simulink library "GOcontroll_Moduline_Target"  (R2018b)
settings: Solver=ode45  StartTime=0.0  StopTime=10.0  RelTol=1e-3  EnableMultiTasking=on
(part 2 of 3)

== system GOcontroll_Moduline_Target/Modules/Input Module ==
  Input Module (10 channel) : Subsystem  Tag=HANcoder_GOcontroll_Moduline_IV  mask(Input Module){tsamp=0.1, ContrType=GOcontroll Moduline IV, moduleSlot=Moduleslot 1, SensSup1=Supply output enabled, C1func=Analog input -  decimal (12 bit resolution), C1pu=no pull up, C1pd=no pull down, C2func=Analog input -  decimal (12 bit resolution), C2pu=no pull up, C2pd=no pull down, C3func=Analog input -  decimal (12 bit resolution), C3pu=no pull up, C3pd=no pull down, C4func=Analog input -  decimal (12 bit resolution), C4pu=no pull up, C4pd=no pull down, C5func=Analog input -  decimal (12 bit resolution), C5pu=no pull up, C5pd=no pull down, C6func=Analog input -  decimal (12 bit resolution), C6pu=no pull up, C6pd=no pull down, C7func=Analog input -  decimal (12 bit resolution), C7pu=no pull up, C7pd=no pull down, C8func=Analog input -  decimal (12 bit resolution), C8pu=no pull up, C8pd=no pull down, C9func=Analog input -  decimal (12 bit resolution), C9pu=no pull up, C9pd=no pull down, C10func=Analog input -  decimal (12 bit resolution), C10pu=no pull up, C10pd=no pull down}
      mask prompts: tsamp "Sample time"; ContrType "Controller Type"; moduleSlot "Module Slot"; SensSup1 "5V Sensor Supply 1"; C1func "Function select"; C1pu "Pull up on input"; C1pd "Pull down on input"; C2func "Function select"; C2pu "Pull up on input"; C2pd "Pull down on input"; C3func "Function select"; C3pu "Pull up on input"; C3pd "Pull down on input"; C4func "Function select"; C4pu "Pull up on input"; C4pd "Pull down on input"; C5func "Function select"; C5pu "Pull up on input"; C5pd "Pull down on input"; C6func "Function select"; C6pu "Pull up on input"; C6pd "Pull down on input"; C7func "Function select"; C7pu "Pull up on input"; C7pd "Pull down on input"; C8func "Function select"; C8pu "Pull up on input"; C8pd "Pull down on input"; C9func "Function select"; C9pu "Pull up on input"; C9pd "Pull down on input"; C10func "Function select"; C10pu "Pull up on input"; C10pd "Pull down on input"
      mask help:
      | Whit this function block, you can configure each channel of the 6 channel input module (201001xx). The configuration of the module is executed once so the input module acts acording the setting. During runtime, the block outputs give the measured values from eacht measured channel which can directly be used inside the model.
      |
      | Module location:
      | Sets the location of the module slot where the module is physically
      | plugged into.
      |
      | Channel tabs:
      | Each channel has its own configuration tab.
      |
      | Function select:
      | Select the desired input signal configuration.
      |
      | Voltage range:
      | Select the expected input range of the signal.
      |
      | Analog filter samples:
      | The number of samples that are passed into a moving average filter.
      | (only active in case of an analog input)
      |
      | Pulses per rotation
      | The number of pulses for one rotation. This parameter is needed in case the
      | module needs to calculate the rotation speed from i.e. an axle.
      |
      | Pull Up:
      | If required, a pull-up resistance can be added to the input signal.
      |
      | Pull Down:
      | If required, a pull-down resistance can be added to the input signal.
      mask init:
      | [moduleSlotInfoStr, connectorId, pin1Id, pin2Id, pin3Id, pin4Id, pin5Id, pin6Id, pin7Id, pin8Id, pin9Id, pin10Id] = sfcn_gocontroll_input_module_10_mcb(moduleSlot,ContrType,C1func,C1pu,C1pd,...
      |                                                             C2func,C2pu,C2pd,...
      | 															C3func,C3pu,C3pd,...
      | 															C4func,C4pu,C4pd,...
      | 															C5func,C5pu,C5pd,...
      | 															C6func,C6pu,C6pd,...
      |                                                             C7func,C7pu,C7pd,...
      |                                                             C8func,C8pu,C8pd,...
      |                                                             C9func,C9pu,C9pd,...
      |                                                             C10func,C10pu,C10pd,...
      |                                                             SensSup1);
      settings: MoveFcn=%%drawLogos
      mask TypeOptions ContrType: GOcontroll Moduline IV | GOcontroll Moduline Mini | GOcontroll Moduline Display
      mask Callback ContrType:
      | msk = Simulink.Mask.get(gcb);
      | p = msk.Parameters;
      | 
      | func = get_param(gcb,'ContrType');
      | 
      | if(func == "GOcontroll Moduline IV")
      | p(3).TypeOptions = {'Moduleslot 1','Moduleslot 2','Moduleslot 3','Moduleslot 4',...
      |                     'Moduleslot 5','Moduleslot 6','Moduleslot 7','Moduleslot 8'};
      | elseif (func == "GOcontroll Moduline Mini")
      |  p(3).TypeOptions = {'Moduleslot 1','Moduleslot 2','Moduleslot 3','Moduleslot 4'};
      | 
      | else (func == "GOcontroll Moduline Screen")
      | p(3).TypeOptions = {'Moduleslot 1','Moduleslot 2'};
      | end
      mask TypeOptions moduleSlot: Moduleslot 1 | Moduleslot 2 | Moduleslot 3 | Moduleslot 4 | Moduleslot 5 | Moduleslot 6 | Moduleslot 7 | Moduleslot 8
      mask TypeOptions SensSup1: Supply output enabled | Supply output disabled
      mask TypeOptions C1func: Analog input -  decimal (12 bit resolution) | Analog input -  mV (1mV resolution) | Digital input - status (high or low) | Digital input - frequency (1Hz to 10 kHz) | Digital input - duty cycle low time (0.1% resolution) | Digital input - dutycycle high time (0.1% resolution) | Digital input - rotation speed (rpm) | Digital input - pulse counter (in combination with channel 2)
      mask TypeOptions C1pu: no pull up | 3,3 K ohm
      mask TypeOptions C1pd: no pull down | 3,3 K ohm
      mask TypeOptions C2func: Analog input -  decimal (12 bit resolution) | Analog input -  mV (1mV resolution) | Digital input - status (high or low) | Digital input - frequency (1Hz to 10 kHz) | Digital input - duty cycle low time (0.1% resolution) | Digital input - dutycycle high time (0.1% resolution) | Digital input - rotation speed (rpm) | Digital input - pulse counter (in combination with channel 2)
      mask TypeOptions C2pu: no pull up | 3,3 K ohm
      mask TypeOptions C2pd: no pull down | 3,3 K ohm
      mask TypeOptions C3func: Analog input -  decimal (12 bit resolution) | Analog input -  mV (1mV resolution) | Digital input - status (high or low) | Digital input - frequency (1Hz to 10 kHz) | Digital input - duty cycle low time (0.1% resolution) | Digital input - dutycycle high time (0.1% resolution) | Digital input - rotation speed (rpm) | Digital input - pulse counter (in combination with channel 2)
      mask TypeOptions C3pu: no pull up | 3,3 K ohm
      mask TypeOptions C3pd: no pull down | 3,3 K ohm
      mask TypeOptions C4func: Analog input -  decimal (12 bit resolution) | Analog input -  mV (1mV resolution) | Digital input - status (high or low) | Digital input - frequency (1Hz to 10 kHz) | Digital input - duty cycle low time (0.1% resolution) | Digital input - dutycycle high time (0.1% resolution) | Digital input - rotation speed (rpm) | Digital input - pulse counter (in combination with channel 2) | TFmini plus - Benewake LIDAR sensor
      mask TypeOptions C4pu: no pull up | 3,3 K ohm
      mask TypeOptions C4pd: no pull down | 3,3 K ohm
      mask TypeOptions C5func: Analog input -  decimal (12 bit resolution) | Analog input -  mV (1mV resolution) | Digital input - status (high or low) | Digital input - frequency (1Hz to 10 kHz) | Digital input - duty cycle low time (0.1% resolution) | Digital input - dutycycle high time (0.1% resolution) | Digital input - rotation speed (rpm) | Digital input - pulse counter (in combination with channel 2)
      mask TypeOptions C5pu: no pull up | 3,3 K ohm
      mask TypeOptions C5pd: no pull down | 3,3 K ohm
      mask TypeOptions C6func: Analog input -  decimal (12 bit resolution) | Analog input -  mV (1mV resolution) | Digital input - status (high or low) | Digital input - frequency (1Hz to 10 kHz) | Digital input - duty cycle low time (0.1% resolution) | Digital input - dutycycle high time (0.1% resolution) | Digital input - rotation speed (rpm) | Digital input - pulse counter (in combination with channel 2)
      mask TypeOptions C6pu: no pull up | 3,3 K ohm
      mask TypeOptions C6pd: no pull down | 3,3 K ohm
      mask TypeOptions C7func: Analog input -  decimal (12 bit resolution) | Analog input -  mV (1mV resolution) | Digital input - status (high or low) | Digital input - frequency (1Hz to 10 kHz) | Digital input - duty cycle low time (0.1% resolution) | Digital input - dutycycle high time (0.1% resolution) | Digital input - rotation speed (rpm) | Digital input - pulse counter (in combination with channel 2)
      mask TypeOptions C7pu: no pull up | 3,3 K ohm
      mask TypeOptions C7pd: no pull down | 3,3 K ohm
      mask TypeOptions C8func: Analog input -  decimal (12 bit resolution) | Analog input -  mV (1mV resolution) | Digital input - status (high or low) | Digital input - frequency (1Hz to 10 kHz) | Digital input - duty cycle low time (0.1% resolution) | Digital input - dutycycle high time (0.1% resolution) | Digital input - rotation speed (rpm) | Digital input - pulse counter (in combination with channel 2)
      mask TypeOptions C8pu: no pull up | 3,3 K ohm
      mask TypeOptions C8pd: no pull down | 3,3 K ohm
      mask TypeOptions C9func: Analog input -  decimal (12 bit resolution) | Analog input -  mV (1mV resolution) | Digital input - status (high or low) | Digital input - frequency (1Hz to 10 kHz) | Digital input - duty cycle low time (0.1% resolution) | Digital input - dutycycle high time (0.1% resolution) | Digital input - rotation speed (rpm) | Digital input - pulse counter (in combination with channel 2) | TFmini plus - Benewake LIDAR sensor
      mask TypeOptions C9pu: no pull up | 3,3 K ohm
      mask TypeOptions C9pd: no pull down | 3,3 K ohm
      mask TypeOptions C10func: Analog input -  decimal (12 bit resolution) | Analog input -  mV (1mV resolution) | Digital input - status (high or low) | Digital input - frequency (1Hz to 10 kHz) | Digital input - duty cycle low time (0.1% resolution) | Digital input - dutycycle high time (0.1% resolution) | Digital input - rotation speed (rpm) | Digital input - pulse counter (in combination with channel 2)
      mask TypeOptions C10pu: no pull up | 3,3 K ohm
      mask TypeOptions C10pd: no pull down | 3,3 K ohm
      mask DialogControl Container4 Prompt: Input 1
      mask DialogControl Container5 Prompt: Input 2
      mask DialogControl Container8 Prompt: Input 3
      mask DialogControl Container9 Prompt: Input 4
      mask DialogControl Container7 Prompt: Input 5
      mask DialogControl Container12 Prompt: Input 6
      mask DialogControl Container6 Prompt: Input 7
      mask DialogControl Container10 Prompt: Input 8
      mask DialogControl Container11 Prompt: Input 9
      mask DialogControl Container13 Prompt: Input 10
      mask Display:
      | fprintf('10 Channel Input Module \n%s\n\n Controller Connector: %s', moduleSlotInfoStr,connectorId);
      | port_label('output', 1, pin1Id);
      | port_label('output', 2, pin2Id);
      | port_label('output', 3, pin3Id);
      | port_label('output', 4, pin4Id);
      | port_label('output', 5, pin5Id);
      | port_label('output', 6, pin6Id);
      | port_label('output', 7, pin7Id);
      | port_label('output', 8, pin8Id);
      | port_label('output', 9, pin9Id);
      | port_label('output', 10, pin10Id);
      | text(2, 6, ert_linux_target_version());
  Input Module (6 channel) : Subsystem  Tag=HANcoder_GOcontroll_Moduline_IV  mask(Input Module){tsamp=0.1, ContrType=GOcontroll Moduline IV, moduleSlot=Moduleslot 1, SensSup1=Supply output enabled, SensSup2=Supply output enabled, SensSup3=Supply output enabled, C1func=Analog input -  decimal (12 bit resolution), C1volt=0 - 5 V, C1afil=0, C1dpul=1, C1pu=no pull up, C1pd=no pull down, C2func=Analog input -  decimal (12 bit resolution), C2volt=0 - 5 V, C2afil=0, C2dpul=1, C2pu=no pull up, C2pd=no pull down, C3func=Analog input -  decimal (12 bit resolution), C3volt=0 - 5 V, C3afil=0, C3dpul=1, C3pu=no pull up, C3pd=no pull down, C4func=Analog input -  decimal (12 bit resolution), C4volt=0 - 5 V, C4afil=0, C4dpul=1, C4pu=no pull up, C4pd=no pull down, C5func=Analog input -  decimal (12 bit resolution), C5volt=0 - 5 V, C5afil=0, C5dpul=1, C5pu=no pull up, C5pd=no pull down, C6func=Analog input -  decimal (12 bit resolution), C6volt=0 - 5 V, C6afil=0, C6dpul=1, C6pu=no pull up, C6pd=no pull down}
      mask prompts: tsamp "Sample time"; ContrType "Controller Type"; moduleSlot "Module Slot"; SensSup1 "5V Sensor Supply 1"; SensSup2 "5V Sensor Supply 2"; SensSup3 "5V Sensor Supply 3"; C1func "Function select"; C1volt "Voltage range"; C1afil "Analog filter samples (0 - 1000)"; C1dpul "Pulses per rotation (1-200)"; C1pu "Pull up on input"; C1pd "Pull down on input"; C2func "Function select"; C2volt "Voltage range"; C2afil "Analog filter samples (0 - 1000)"; C2dpul "Pulses per rotation (1-200)"; C2pu "Pull up on input"; C2pd "Pull down on input"; C3func "Function select"; C3volt "Voltage range"; C3afil "Analog filter samples (0 - 1000)"; C3dpul "Pulses per rotation (1-200)"; C3pu "Pull up on input"; C3pd "Pull down on input"; C4func "Function select"; C4volt "Voltage range"; C4afil "Analog filter samples (0 - 1000)"; C4dpul "Pulses per rotation (1-200)"; C4pu "Pull up on input"; C4pd "Pull down on input"; C5func "Function select"; C5volt "Voltage range"; C5afil "Analog filter samples (0 - 1000)"; C5dpul "Pulses per rotation (1-200)"; C5pu "Pull up on input"; C5pd "Pull down on input"; C6func "Function select"; C6volt "Voltage range"; C6afil "Analog filter samples (0 - 1000)"; C6dpul "Pulses per rotation (1-200)"; C6pu "Pull up on input"; C6pd "Pull down on input"
      mask help:
      | Whit this function block, you can configure each channel of the 6 channel input module (201001xx). The configuration of the module is executed once so the input module acts acording the setting. During runtime, the block outputs give the measured values from eacht measured channel which can directly be used inside the model.
      |
      | Module location:
      | Sets the location of the module slot where the module is physically
      | plugged into.
      |
      | Channel tabs:
      | Each channel has its own configuration tab.
      |
      | Function select:
      | Select the desired input signal configuration.
      |
      | Voltage range:
      | Select the expected input range of the signal.
      |
      | Analog filter samples:
      | The number of samples that are passed into a moving average filter.
      | (only active in case of an analog input)
      |
      | Pulses per rotation
      | The number of pulses for one rotation. This parameter is needed in case the
      | module needs to calculate the rotation speed from i.e. an axle.
      |
      | Pull Up:
      | If required, a pull-up resistance can be added to the input signal.
      |
      | Pull Down:
      | If required, a pull-down resistance can be added to the input signal.
      mask init:
      | [moduleSlotInfoStr, connectorId, pin1Id, pin2Id, pin3Id, pin4Id, pin5Id, pin6Id] = sfcn_gocontroll_input_module_mcb(moduleSlot,ContrType, C1func,C1volt,C1afil,C1dpul,C1pu,C1pd,...
      |                                                             C2func,C2volt,C2afil,C2dpul,C2pu,C2pd,...
      | 															C3func,C3volt,C3afil,C3dpul,C3pu,C3pd,...
      | 															C4func,C4volt,C4afil,C4dpul,C4pu,C4pd,...
      | 															C5func,C5volt,C5afil,C5dpul,C5pu,C5pd,...
      | 															C6func,C6volt,C6afil,C6dpul,C6pu,C6pd,...
      |                                                             SensSup1,SensSup2,SensSup3);
      settings: MoveFcn=%%drawLogos
      mask TypeOptions ContrType: GOcontroll Moduline IV | GOcontroll Moduline Mini | GOcontroll Moduline Display
      mask Callback ContrType:
      | msk = Simulink.Mask.get(gcb);
      | p = msk.Parameters;
      | 
      | func = get_param(gcb,'ContrType');
      | 
      | if(func == "GOcontroll Moduline IV")
      | p(3).TypeOptions = {'Moduleslot 1','Moduleslot 2','Moduleslot 3','Moduleslot 4',...
      |                     'Moduleslot 5','Moduleslot 6','Moduleslot 7','Moduleslot 8'};
      | elseif (func == "GOcontroll Moduline Mini")
      |  p(3).TypeOptions = {'Moduleslot 1','Moduleslot 2','Moduleslot 3','Moduleslot 4'};
      | 
      | else (func == "GOcontroll Moduline Screen")
      | p(3).TypeOptions = {'Moduleslot 1','Moduleslot 2'};
      | end
      mask TypeOptions moduleSlot: Moduleslot 1 | Moduleslot 2 | Moduleslot 3 | Moduleslot 4 | Moduleslot 5 | Moduleslot 6 | Moduleslot 7 | Moduleslot 8
      mask TypeOptions SensSup1: Supply output enabled | Supply output disabled
      mask TypeOptions SensSup2: Supply output enabled | Supply output disabled
      mask TypeOptions SensSup3: Supply output enabled | Supply output disabled
      mask TypeOptions C1func: Analog input -  decimal (12 bit resolution) | Analog input -  mV (1mV resolution) | Digital input - status (high or low) | Digital input - frequency (1Hz to 10 kHz) | Digital input - duty cycle low time (0.1% resolution) | Digital input - dutycycle high time (0.1% resolution) | Digital input - rotation speed (rpm) | Digital input - pulse counter (in combination with channel 2)
      mask TypeOptions C1volt: 0 - 5 V | 0 - 10V (external sensor supply) | 0 - 24V (external sensor supply)
      mask TypeOptions C1pu: no pull up | 3,3 K ohm | 4,7 K ohm | 10 K ohm
      mask TypeOptions C1pd: no pull down | 3,3 K ohm | 4,7 K ohm | 10 K ohm
      mask TypeOptions C2func: Analog input -  decimal (12 bit resolution) | Analog input -  mV (1mV resolution) | Digital input - status (high or low) | Digital input - frequency (1Hz to 10 kHz) | Digital input - duty cycle low time (0.1% resolution) | Digital input - dutycycle high time (0.1% resolution) | Digital input - rotation speed (rpm) | Digital input - pulse counter (in combination with channel 2)
      mask TypeOptions C2volt: 0 - 5 V | 0 - 10V (external sensor supply) | 0 - 24V (external sensor supply)
      mask TypeOptions C2pu: no pull up | 3,3 K ohm | 4,7 K ohm | 10 K ohm
      mask TypeOptions C2pd: no pull down | 3,3 K ohm | 4,7 K ohm | 10 K ohm
      mask TypeOptions C3func: Analog input -  decimal (12 bit resolution) | Analog input -  mV (1mV resolution) | Digital input - status (high or low) | Digital input - frequency (1Hz to 10 kHz) | Digital input - duty cycle low time (0.1% resolution) | Digital input - dutycycle high time (0.1% resolution) | Digital input - rotation speed (rpm) | Digital input - pulse counter (in combination with channel 2)
      mask TypeOptions C3volt: 0 - 5 V | 0 - 10V (external sensor supply) | 0 - 24V (external sensor supply)
      mask TypeOptions C3pu: no pull up | 3,3 K ohm | 4,7 K ohm | 10 K ohm
      mask TypeOptions C3pd: no pull down | 3,3 K ohm | 4,7 K ohm | 10 K ohm
      mask TypeOptions C4func: Analog input -  decimal (12 bit resolution) | Analog input -  mV (1mV resolution) | Digital input - status (high or low) | Digital input - frequency (1Hz to 10 kHz) | Digital input - duty cycle low time (0.1% resolution) | Digital input - dutycycle high time (0.1% resolution) | Digital input - rotation speed (rpm) | Digital input - pulse counter (in combination with channel 2) | TFmini plus - Benewake LIDAR sensor
      mask TypeOptions C4volt: 0 - 5 V | 0 - 10V (external sensor supply) | 0 - 24V (external sensor supply)
      mask TypeOptions C4pu: no pull up | 3,3 K ohm | 4,7 K ohm | 10 K ohm
      mask TypeOptions C4pd: no pull down | 3,3 K ohm | 4,7 K ohm | 10 K ohm
      mask TypeOptions C5func: Analog input -  decimal (12 bit resolution) | Analog input -  mV (1mV resolution) | Digital input - status (high or low) | Digital input - frequency (1Hz to 10 kHz) | Digital input - duty cycle low time (0.1% resolution) | Digital input - dutycycle high time (0.1% resolution) | Digital input - rotation speed (rpm) | Digital input - pulse counter (in combination with channel 2)
      mask TypeOptions C5volt: 0 - 5 V | 0 - 10V (external sensor supply) | 0 - 24V (external sensor supply)
      mask TypeOptions C5pu: no pull up | 3,3 K ohm | 4,7 K ohm | 10 K ohm
      mask TypeOptions C5pd: no pull down | 3,3 K ohm | 4,7 K ohm | 10 K ohm
      mask TypeOptions C6func: Analog input -  decimal (12 bit resolution) | Analog input -  mV (1mV resolution) | Digital input - status (high or low) | Digital input - frequency (1Hz to 10 kHz) | Digital input - duty cycle low time (0.1% resolution) | Digital input - dutycycle high time (0.1% resolution) | Digital input - rotation speed (rpm) | Digital input - pulse counter (in combination with channel 2)
      mask TypeOptions C6volt: 0 - 5 V | 0 - 10V (external sensor supply) | 0 - 24V (external sensor supply)
      mask TypeOptions C6pu: no pull up | 3,3 K ohm | 4,7 K ohm | 10 K ohm
      mask TypeOptions C6pd: no pull down | 3,3 K ohm | 4,7 K ohm | 10 K ohm
      mask DialogControl Container4 Prompt: Input 1
      mask DialogControl Container5 Prompt: Input 2
      mask DialogControl Container8 Prompt: Input 3
      mask DialogControl Container9 Prompt: Input 4
      mask DialogControl Container7 Prompt: Input 5
      mask DialogControl Container12 Prompt: Input 6
      mask Display:
      | fprintf('6 Channel Input Module \n%s\n\n Controller Connector: %s', moduleSlotInfoStr,connectorId);
      | port_label('output', 1, pin1Id);
      | port_label('output', 2, pin2Id);
      | port_label('output', 3, pin3Id);
      | port_label('output', 4, pin4Id);
      | port_label('output', 5, pin5Id);
      | port_label('output', 6, pin6Id);
      | text(2, 6, ert_linux_target_version());
  Input Module 4-20 mA (10 channel) : Subsystem  Tag=HANcoder_GOcontroll_Moduline_IV  mask(4-20 mA Input Module){tsamp=0.1, ContrType=GOcontroll Moduline IV, moduleSlot=Moduleslot 1, Sup16va=Supply enabled}
      mask prompts: tsamp "Sample time"; ContrType "Controller type"; moduleSlot "Module slot"; Sup16va "16V sensor supply"
      mask help:
      | Controller type:
      | Selects the controller that is to be programmed. Pinning on the mask will be adopted accordingly.
      |
      | Module slot:
      | Sets the location of the module slot where the module is physically plugged into.
      |
      | 16V sensor supply:
      | Enables the 16V supply for all the sensors. When this supply is not enabled possible no current flows through the sensors.
      |
      | Module status:
      | The status output provides information of the actual state per 2 channels:
      | 0x00 all channels are supplied no problems.
      | 0x01Channel 1 & 2 over current detected and supply disconnected.
      | 0x02Channel 3 & 4 over current detected and supply disconnected.
      | 0x04Channel 5 & 6 over current detected and supply disconnected.
      | 0x08Channel 7 & 8 over current detected and supply disconnected.
      | 0x10Channel 9 & 10 over current detected and supply disconnected.
      mask init:
      | [moduleSlotInfoStr, connectorId, pin1Id, pin2Id, pin3Id, pin4Id, pin5Id, pin6Id, pin7Id, pin8Id, pin9Id, pin10Id] =...
      |     sfcn_gocontroll_input_module_420ma_mcb(moduleSlot,ContrType,Sup16va);
      settings: MoveFcn=%%drawLogos
      mask TypeOptions ContrType: GOcontroll Moduline IV | GOcontroll Moduline Mini | GOcontroll Moduline Display
      mask Callback ContrType:
      | msk = Simulink.Mask.get(gcb);
      | p = msk.Parameters;
      | 
      | func = get_param(gcb,'ContrType');
      | 
      | if(func == "GOcontroll Moduline IV")
      | p(3).TypeOptions = {'Moduleslot 1','Moduleslot 2','Moduleslot 3','Moduleslot 4',...
      |                     'Moduleslot 5','Moduleslot 6','Moduleslot 7','Moduleslot 8'};
      | elseif (func == "GOcontroll Moduline Mini")
      |  p(3).TypeOptions = {'Moduleslot 1','Moduleslot 2','Moduleslot 3','Moduleslot 4'};
      | 
      | else (func == "GOcontroll Moduline Screen")
      | p(3).TypeOptions = {'Moduleslot 1','Moduleslot 2'};
      | end
      mask TypeOptions moduleSlot: Moduleslot 1 | Moduleslot 2 | Moduleslot 3 | Moduleslot 4 | Moduleslot 5 | Moduleslot 6 | Moduleslot 7 | Moduleslot 8
      mask TypeOptions Sup16va: Supply disabled | Supply enabled
      mask Display:
      | fprintf('4-20 mA Input Module \n%s\n\n Controller Connector: %s', moduleSlotInfoStr,connectorId);
      | port_label('output', 1, "Status");
      | port_label('output', 2, pin1Id);
      | port_label('output', 3, pin2Id);
      | port_label('output', 4, pin3Id);
      | port_label('output', 5, pin4Id);
      | port_label('output', 6, pin5Id);
      | port_label('output', 7, pin6Id);
      | port_label('output', 8, pin7Id);
      | port_label('output', 9, pin8Id);
      | port_label('output', 10, pin9Id);
      | port_label('output', 11, pin10Id);
      | text(2, 6, ert_linux_target_version());
  Reset Puls Counter (6 channel) : Subsystem  Tag=HANcoder_GOcontroll_Moduline_IV  mask(Reset puls counter){tsamp=-1, contrType=GOcontroll Moduline IV, moduleSlot=Moduleslot 1, channel=Reset pulscounter on channel 1}
      mask prompts: tsamp "Sample time"; contrType "Controller Type"; moduleSlot "Module slot"
      mask help: This function block resets the pulscounter from a specified input channel of the input module that is configured as a pulscounter. A trigger on input pin 1 wil set the pulscounter to the value applied on pin 2
      mask init:
      | [moduleSlotInfoStr, inputChannelInfoStr] = sfcn_gocontroll_input_module_reset_mcb(moduleSlot,contrType,channel);
      mask TypeOptions contrType: GOcontroll Moduline IV | GOcontroll Moduline Mini | GOcontroll Moduline Display
      mask Callback contrType:
      | msk = Simulink.Mask.get(gcb);
      | p = msk.Parameters;
      | 
      | func = get_param(gcb,'ContrType');
      | 
      | if(func == "GOcontroll Moduline IV")
      | p(3).TypeOptions = {'Moduleslot 1','Moduleslot 2','Moduleslot 3','Moduleslot 4',...
      |                     'Moduleslot 5','Moduleslot 6','Moduleslot 7','Moduleslot 8'};
      | elseif (func == "GOcontroll Moduline Mini")
      |  p(3).TypeOptions = {'Moduleslot 1','Moduleslot 2','Moduleslot 3','Moduleslot 4'};
      | 
      | elseif (func == "GOcontroll Moduline Screen")
      |  p(3).TypeOptions = {'Moduleslot 1','Moduleslot 2'};
      | end
      mask TypeOptions moduleSlot: Moduleslot 1 | Moduleslot 2 | Moduleslot 3 | Moduleslot 4 | Moduleslot 5 | Moduleslot 6 | Moduleslot 7 | Moduleslot 8
      mask TypeOptions channel: Reset pulscounter on channel 1 | Reset pulscounter on channel 2 | Reset pulscounter on channel 3 | Reset pulscounter on channel 4 | Reset pulscounter on channel 5 | Reset pulscounter on channel 6
      mask Display:
      | fprintf('Reset Puls Counter\n%s\n%s', moduleSlotInfoStr, inputChannelInfoStr);
      | text(2, 6, ert_linux_target_version());
